simulink model "lab7"  (R2023b)
settings: Solver=ode45  StartTime=0.0  StopTime=15  MaxStep=2^(-5)  RelTol=1e-3
settings Model: Creator=insomnia  LastModifiedBy=insomnia

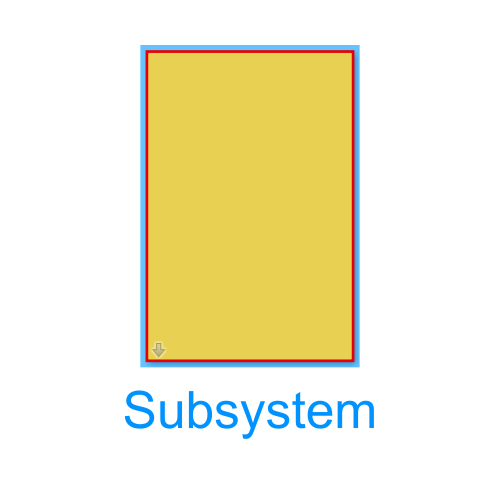
[thumbnail: Simulink's stored preview of the top-level diagram]
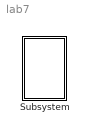
== system lab7 ==
  Subsystem : Subsystem  mask{g=9.81, k1=2, k2=1, m1=1, m2=2, l1=1, l2=2, th10=80, th20=150, th11=0, th21=0}
      mask prompts: g "przyspieszenie ziemskie"; k1 "wsp. tlumienia 1"; k2 "wsp. tlumienia 2"; m1 "masa 1"; m2 "masa 2"; l1 "dlugosc linki 1"; l2 "dlugosc linki 2"; th10 "kat wychylenia 1"; th20 "kat wychylenia 2"; th11 "predkosc wahadla 1"; th21 "predkosc wahadla 2"

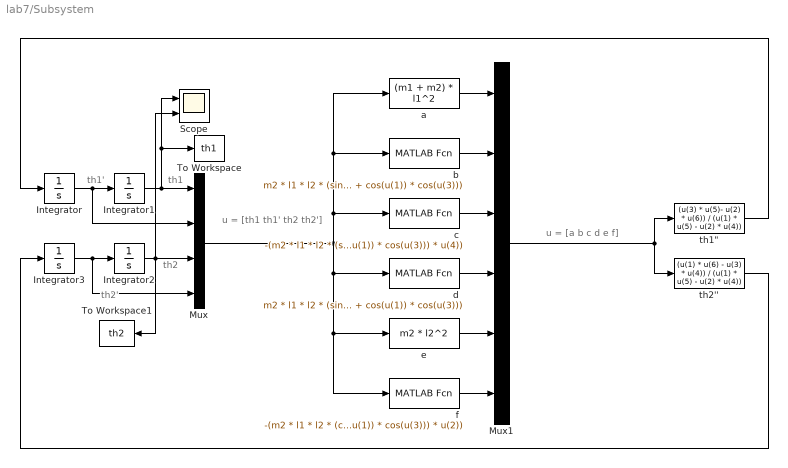
== system lab7/Subsystem ==
  note: th1'
  note: u = [th1 th1' th2 th2']
  note: th2'
  note: th1
  note: u = [a b c d e f]
  note: th2
  Integrator : Integrator  InitialCondition=th11 * pi/180
  Integrator1 : Integrator  InitialCondition=th10 * pi/180
  Integrator2 : Integrator  InitialCondition=th20 * pi / 180
  Integrator3 : Integrator  InitialCondition=th21 * pi / 180
  Mux : Mux
  Mux1 : Mux  Inputs=6
  Scope : Scope  NumInputPorts=2
  To Workspace : ToWorkspace  VariableName=th1  SampleTime=-1
  To Workspace1 : ToWorkspace  VariableName=th2  SampleTime=-1
  a : MATLABFcn  MATLABFcn=(m1 + m2) * l1^2
  b : MATLABFcn  MATLABFcn=m2 * l1 * l2 * (sin(u(1)) * sin(u(3)) + cos(u(1)) * cos(u(3)))
  c : MATLABFcn  MATLABFcn=-(m2 * l1 * l2 * (sin(u(1)) * cos(u(3)) - cos(u(1)) * sin(u(3))) * u(4)^2 + (m1 + m2) * g * l1 * sin(u(1)) + k1 * l1^2 * u(2) + k2 * l1 * l2 * (sin(u(1)) * sin(u(3)) + cos(u(1)) * cos(u(3))) * u(4))
  d : MATLABFcn  MATLABFcn=m2 * l1 * l2 * (sin(u(1)) * sin(u(3)) + cos(u(1)) * cos(u(3)))
  e : MATLABFcn  MATLABFcn=m2 * l2^2
  f : MATLABFcn  MATLABFcn=-(m2 * l1 * l2 * (cos(u(1)) * sin(u(3)) - sin(u(1)) * cos(u(3))) * u(2)^2 + m2 * g * l2 * sin(u(3)) + k2 * l2^2 * u(4) + k2 * l1 * l2 * (sin(u(1)) * sin(u(3)) + cos(u(1)) * cos(u(3))) * u(2))
  "th1\"" : MATLABFcn  MATLABFcn=(u(3) * u(5)- u(2) * u(6)) / (u(1) * u(5) - u(2) * u(4))
  th2'' : MATLABFcn  MATLABFcn=(u(1) * u(6) - u(3) * u(4)) / (u(1) * u(5) - u(2) * u(4))
  wires:
  Integrator/1 -> Mux/2, Integrator1/1
  Mux1/1 -> "th1\""/1, th2''/1
  "th1\""/1 -> Integrator/1
  e/1 -> Mux1/5
  Integrator2/1 -> Scope/2, To Workspace1/1, Mux/3
  Integrator3/1 -> Mux/4, Integrator2/1
  d/1 -> Mux1/4
  th2''/1 -> Integrator3/1
  Mux/1 -> a/1, b/1, c/1, f/1, e/1, d/1
  a/1 -> Mux1/1
  f/1 -> Mux1/6
  Integrator1/1 -> To Workspace/1, Scope/1, Mux/1
  c/1 -> Mux1/3
  b/1 -> Mux1/2
